simulink model "BSD_Diagnostic_SWC"  (R2024a)
settings: Solver=FixedStepDiscrete  StartTime=0.0  StopTime=10.0  FixedStep=0.1  RelTol=1e-3
settings Model: Creator=pc  LastModifiedBy=pc
settings OptimizationCC: DefaultParameterBehavior=Inlined  EnhancedBackFolding=on  PassReuseOutputArgsAs=Individual arguments  ZeroExternalMemoryAtStartup=off  ZeroInternalMemoryAtStartup=off  OptimizeBlockOrder=speed  DifferentSizesBufferReuse=on  OptimizationCustomize=off  EfficientTunableParamExpr=on
settings DebuggingCC: ParameterTunabilityLossMsg=error
settings SFSimCC: MATLABDynamicMemAlloc=off
settings RTWCC: Description=AUTOSAR  SystemTargetFile=autosar.tlc  GenCodeOnly=on  TemplateMakefile=ert_default_tmf  GenerateReport=on  LaunchReport=on  DataTypeReplacement=CDataTypesFixedWidth  GenerateWebview=on  GenerateCodeMetricsReport=on
settings CodeAppCC: ForceParamTrailComments=on  IgnoreCustomStorageClasses=off  OperatorAnnotations=on  SimulinkDataObjDesc=on  SFDataObjDesc=on  InsertBlockDesc=on
settings STFCustomTargetCC: MultiwordLength=256  ParMdlRefBuildCompliant=on  CompOptLevelCompliant=on  IncludeMdlTerminateFcn=off  CombineOutputUpdateFcns=on  SuppressErrorStatus=on  ERTCustomFileBanners=on  SupportNonFinite=off  SupportComplex=off  SupportContinuousTime=off  SupportNonInlinedSFcns=off  RemoveResetFunc=on  MATLABClassNameForMDSCustomization=Simulink.SoftwareTarget.ERTCustomization  AutosarCompliant=on  GRTInterface=off  LookupTableObjectStructAxisOrder=2,1,3,4,...  LUTObjectStructOrderEvenSpacing=Size,Table,Breakpoints  SystemTargetFile=autosar.tlc
settings ERTTargetCC: TargetLangStandard=C99 (ISO)  ConcurrentExecutionCompliant=off  IncludeMdlTerminateFcn=off  SuppressErrorStatus=on  SupportNonFinite=off  SupportComplex=off  ModelStepFunctionPrototypeControlCompliant=off  CPPClassGenCompliant=off  AutosarCompliant=on  LookupTableObjectStructAxisOrder=2,1,3,4,...  LUTObjectStructOrderEvenSpacing=Size,Table,Breakpoints  InlinedParameterPlacement=NonHierarchical  ERTCustomFileTemplate=example_file_process.tlc  BooleanTrueId=TRUE  BooleanFalseId=FALSE

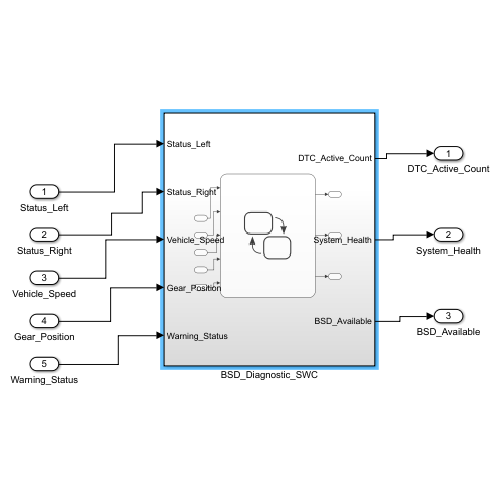
[thumbnail: Simulink's stored preview of the top-level diagram]
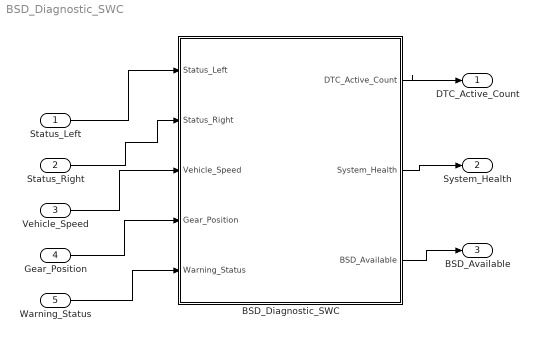
== system BSD_Diagnostic_SWC ==
  Status_Left : Inport  OutDataTypeStr=uint8
  Status_Right : Inport  Port=2  OutDataTypeStr=uint8
  Vehicle_Speed : Inport  Port=3  OutDataTypeStr=single
  Gear_Position : Inport  Port=4  OutDataTypeStr=uint8
  Warning_Status : Inport  Port=5  OutDataTypeStr=uint8
  BSD_Diagnostic_SWC : Subsystem
  DTC_Active_Count : Outport  OutDataTypeStr=uint8
  System_Health : Outport  Port=2  OutDataTypeStr=uint8
  BSD_Available : Outport  Port=3  OutDataTypeStr=uint8
  wires:
  Status_Left/1 -> BSD_Diagnostic_SWC/1(Status_Left)
  Status_Right/1 -> BSD_Diagnostic_SWC/2(Status_Right)
  Vehicle_Speed/1 -> BSD_Diagnostic_SWC/3(Vehicle_Speed)
  Gear_Position/1 -> BSD_Diagnostic_SWC/4(Gear_Position)
  Warning_Status/1 -> BSD_Diagnostic_SWC/5(Warning_Status)
  BSD_Diagnostic_SWC/1(DTC_Active_Count) -> DTC_Active_Count/1
  BSD_Diagnostic_SWC/3(BSD_Available) -> BSD_Available/1
  BSD_Diagnostic_SWC/2(System_Health) -> System_Health/1

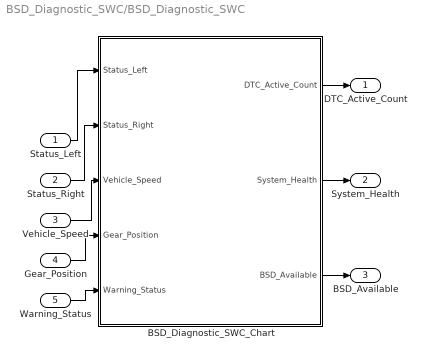
== system BSD_Diagnostic_SWC/BSD_Diagnostic_SWC ==
  Status_Left : Inport
  Status_Right : Inport  Port=2
  Vehicle_Speed : Inport  Port=3
  Gear_Position : Inport  Port=4
  Warning_Status : Inport  Port=5
  BSD_Diagnostic_SWC_Chart : Stateflow chart  TreatAsAtomicUnit=on
      settings: PortSchema="{\"entries\":[{\"content\":{\"sides\":[{\"content\":{\"connectorIds\":[\"In1\",\"In2\",\"In3\",\"In5\",\"In4\"]},\"type\":\"ConnectorPlacement.EquallySpacedRectSide\",\"uuid\":\"c698d591-9237-4f9d-ac39-13ac35c06135\"},{\"content\":{\"connectorIds\":[\"Out1\",\"Out2\",\"Out3\"],\"side\":\"RIGHT\"},\"type\":\"ConnectorPlacement.EquallySpacedRectSide\",\"uuid\":\"e3273571-067e-4dde-a9ad-d8fc7d6bc43a\"},{\"content\":{\"side\":\"TOP\"},\"type\":\"ConnectorPlacement.EquallySpacedRectSide\",\"uuid\":\"59a8224d-d599-4a56-a48e-1dbd2f775c83\"}]},\"type\":\"ConnectorPlacement.EquallySpacedConnector\",\"uuid\":\"096dcc20-cc3f-45af-83ae-7f2277698854\"}],\"packageUris\":[\"http://schema.mathworks.com/mf0/Connector/R2020b\"],\"version\":\"1.0\"}"
  DTC_Active_Count : Outport
  System_Health : Outport  Port=2
  BSD_Available : Outport  Port=3
  wires:
  BSD_Diagnostic_SWC_Chart/1(DTC_Active_Count) -> DTC_Active_Count/1
  BSD_Diagnostic_SWC_Chart/2(System_Health) -> System_Health/1
  BSD_Diagnostic_SWC_Chart/3(BSD_Available) -> BSD_Available/1
  Status_Left/1 -> BSD_Diagnostic_SWC_Chart/1(Status_Left)
  Status_Right/1 -> BSD_Diagnostic_SWC_Chart/2(Status_Right)
  Vehicle_Speed/1 -> BSD_Diagnostic_SWC_Chart/3(Vehicle_Speed)
  Gear_Position/1 -> BSD_Diagnostic_SWC_Chart/5(Gear_Position)
  Warning_Status/1 -> BSD_Diagnostic_SWC_Chart/4(Warning_Status)

== stateflow chart BSD_Diagnostic_SWC/BSD_Diagnostic_SWC_Chart ==
  state SYSTEM_DEGRADED
    entry:
    System_Health = uint8(1);
    BSD_Available = uint8(1);
    during:
    %% ── Debounce Left Sensor ── (replace existing logic)
    if Status_Left ~= uint8(0)          % covers FAIL + BLOCKED + DEGRADED
    Counter_L = Counter_L + uint8(1);
    else
    Counter_L    = uint8(0);
    DTC_L_Active = uint8(0);
    DTC_L_Type   = uint8(0);
    end
    if Counter_L >= uint8(5)
    DTC_L_Active = uint8(1);
    %% Specific DTC type based on status
    if Status_Left == uint8(1)
    DTC_L_Type = uint8(1);       % FAIL
    elseif Status_Left == uint8(2)
    DTC_L_Type = uint8(2);       % BLOCKED
    else
    DTC_L_Type = uint8(3);       % DEGRADED
    end
    Counter_L = uint8(5);
    end
    %% ── Same for Right ──
    if Status_Right ~= uint8(0)
    Counter_R = Counter_R + uint8(1);
    else
    Counter_R    = uint8(0);
    DTC_R_Active = uint8(0);
    DTC_R_Type   = uint8(0);
    end
    if Counter_R >= uint8(5)
    DTC_R_Active = uint8(1);
    %% ── ADD THIS BLOCK ──
    if Status_Right == uint8(1)
    DTC_R_Type = uint8(1);       % FAIL
    elseif Status_Right == uint8(2)
    DTC_R_Type = uint8(2);       % BLOCKED
    else
    DTC_R_Type = uint8(3);       % DEGRADED
    end
    Counter_R = uint8(5);
    end
    %% ── Debounce Speed Signal ──
    if Vehicle_Speed <= single(0.5) && Gear_Position == uint8(3)
    Counter_Speed = Counter_Speed + uint8(1);
    else
    Counter_Speed    = uint8(0);
    DTC_Speed_Active = uint8(0);
    end
    if Counter_Speed >= uint8(10)     % 10 cycles × 100ms = 1 sec
    DTC_Speed_Active = uint8(1);
    Counter_Speed    = uint8(10);
    end
    %% ── DTC_SYSTEM_DEGRADED Detection ──
    %% Triggered when: warning active BUT sensor is degraded quality
    if (Warning_Status > uint8(0)) && (Status_Left == uint8(3) || Status_Right == uint8(3))
    DTC_Degraded_Active = uint8(1);
    else
    DTC_Degraded_Active = uint8(0);
    end
    %% ── Count Active DTCs ──
    DTC_Active_Count = DTC_L_Active + DTC_R_Active +  DTC_Speed_Active + DTC_Degraded_Active;
  state SYSTEM_OK
    entry:
    System_Health    = uint8(0);
    BSD_Available    = uint8(1);
    during:
    %% ── Debounce Left Sensor ── (replace existing logic)
    if Status_Left ~= uint8(0)          % covers FAIL + BLOCKED + DEGRADED
    Counter_L = Counter_L + uint8(1);
    else
    Counter_L    = uint8(0);
    DTC_L_Active = uint8(0);
    DTC_L_Type   = uint8(0);
    end
    if Counter_L >= uint8(5)
    DTC_L_Active = uint8(1);
    %% Specific DTC type based on status
    if Status_Left == uint8(1)
    DTC_L_Type = uint8(1);       % FAIL
    elseif Status_Left == uint8(2)
    DTC_L_Type = uint8(2);       % BLOCKED
    else
    DTC_L_Type = uint8(3);       % DEGRADED
    end
    Counter_L = uint8(5);
    end
    %% ── Same for Right ──
    if Status_Right ~= uint8(0)
    Counter_R = Counter_R + uint8(1);
    else
    Counter_R    = uint8(0);
    DTC_R_Active = uint8(0);
    DTC_R_Type   = uint8(0);
    end
    if Counter_R >= uint8(5)
    DTC_R_Active = uint8(1);
    %% ── ADD THIS BLOCK ──
    if Status_Right == uint8(1)
    DTC_R_Type = uint8(1);       % FAIL
    elseif Status_Right == uint8(2)
    DTC_R_Type = uint8(2);       % BLOCKED
    else
    DTC_R_Type = uint8(3);       % DEGRADED
    end
    Counter_R = uint8(5);
    end
    %% ── Debounce Speed Signal ──
    if Vehicle_Speed <= single(0.5) && Gear_Position == uint8(3)
    Counter_Speed = Counter_Speed + uint8(1);
    else
    Counter_Speed    = uint8(0);
    DTC_Speed_Active = uint8(0);
    end
    if Counter_Speed >= uint8(10)     % 10 cycles × 100ms = 1 sec
    DTC_Speed_Active = uint8(1);
    Counter_Speed    = uint8(10);
    end
    %% ── DTC_SYSTEM_DEGRADED Detection ──
    %% Triggered when: warning active BUT sensor is degraded quality
    if (Warning_Status > uint8(0)) && (Status_Left == uint8(3) || Status_Right == uint8(3))
    DTC_Degraded_Active = uint8(1);
    else
    DTC_Degraded_Active = uint8(0);
    end
    %% ── Count Active DTCs ──
    DTC_Active_Count = DTC_L_Active + DTC_R_Active +  DTC_Speed_Active + DTC_Degraded_Active;
  state SYSTEM_FAIL
    entry:
    System_Health = uint8(2);
    BSD_Available = uint8(0);
    during:
    %% ── Debounce Left Sensor ── (replace existing logic)
    if Status_Left ~= uint8(0)          % covers FAIL + BLOCKED + DEGRADED
    Counter_L = Counter_L + uint8(1);
    else
    Counter_L    = uint8(0);
    DTC_L_Active = uint8(0);
    DTC_L_Type   = uint8(0);
    end
    if Counter_L >= uint8(5)
    DTC_L_Active = uint8(1);
    %% Specific DTC type based on status
    if Status_Left == uint8(1)
    DTC_L_Type = uint8(1);       % FAIL
    elseif Status_Left == uint8(2)
    DTC_L_Type = uint8(2);       % BLOCKED
    else
    DTC_L_Type = uint8(3);       % DEGRADED
    end
    Counter_L = uint8(5);
    end
    %% ── Same for Right ──
    if Status_Right ~= uint8(0)
    Counter_R = Counter_R + uint8(1);
    else
    Counter_R    = uint8(0);
    DTC_R_Active = uint8(0);
    DTC_R_Type   = uint8(0);
    end
    if Counter_R >= uint8(5)
    DTC_R_Active = uint8(1);
    %% ── ADD THIS BLOCK ──
    if Status_Right == uint8(1)
    DTC_R_Type = uint8(1);       % FAIL
    elseif Status_Right == uint8(2)
    DTC_R_Type = uint8(2);       % BLOCKED
    else
    DTC_R_Type = uint8(3);       % DEGRADED
    end
    Counter_R = uint8(5);
    end
    %% ── Debounce Speed Signal ──
    if Vehicle_Speed <= single(0.5) && Gear_Position == uint8(3)
    Counter_Speed = Counter_Speed + uint8(1);
    else
    Counter_Speed    = uint8(0);
    DTC_Speed_Active = uint8(0);
    end
    if Counter_Speed >= uint8(10)     % 10 cycles × 100ms = 1 sec
    DTC_Speed_Active = uint8(1);
    Counter_Speed    = uint8(10);
    end
    %% ── DTC_SYSTEM_DEGRADED Detection ──
    %% Triggered when: warning active BUT sensor is degraded quality
    if (Warning_Status > uint8(0)) && (Status_Left == uint8(3) || Status_Right == uint8(3))
    DTC_Degraded_Active = uint8(1);
    else
    DTC_Degraded_Active = uint8(0);
    end
    %% ── Count Active DTCs ──
    DTC_Active_Count = DTC_L_Active + DTC_R_Active +  DTC_Speed_Active + DTC_Degraded_Active;
  (default) -> SYSTEM_OK
  SYSTEM_OK -> SYSTEM_DEGRADED [order 1] : [DTC_Active_Count > uint8(0) &&  ~(DTC_L_Active == uint8(1) && DTC_R_Active == uint8(1))]
  SYSTEM_DEGRADED -> SYSTEM_OK [order 1] : [DTC_Active_Count == uint8(0)]
  SYSTEM_FAIL -> SYSTEM_OK [order 1] : [DTC_Active_Count == uint8(0)]
  SYSTEM_OK -> SYSTEM_FAIL [order 2] : [DTC_L_Active == uint8(1) && DTC_R_Active == uint8(1)]
  SYSTEM_FAIL -> SYSTEM_DEGRADED [order 2] : [DTC_Active_Count > uint8(0) &&  ~(DTC_L_Active == uint8(1) && DTC_R_Active == uint8(1))]
  SYSTEM_DEGRADED -> SYSTEM_FAIL [order 2] : [DTC_L_Active == uint8(1) && DTC_R_Active == uint8(1)]
  data: DTC_Active_Count output uint8 =0; System_Health output uint8 =0; BSD_Available output uint8 =1; Status_Left input uint8; Status_Right input uint8; Vehicle_Speed input single; Warning_Status input uint8; Gear_Position input uint8; Counter_L local uint8 =0; Counter_R local uint8 =0; Counter_Speed local uint8 =0; DTC_L_Active local uint8 =0; DTC_R_Active local uint8 =0; DTC_Speed_Active local uint8 =0; DTC_L_Type local uint8 =0; DTC_R_Type local uint8 =0; DTC_Degraded_Active local uint8 =0
